simulink model "Simulaciones_Practica2"  (R2021b)
settings: Solver=FixedStepAuto  StartTime=0.0  StopTime=40  FixedStep=0.01  RelTol=1e-3
undefined symbols (not defined in the file or in its folder): b, B, den1, den2, denc, denImp, denR1sim, denR2sim, denR3sim, denR4sim, J, K, k, Kb, Kp, L, m, num1, num2, numc, numImp, numR1sim, numR2sim, numR3sim, numR4sim, R, T, T2
libraries: simulink x9, dspsrcs4 x1
settings Model: Creator=e.delpico.2020  LastModifiedBy=Esther

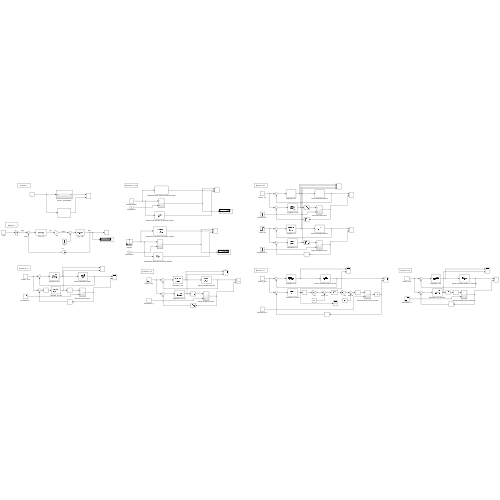
[thumbnail: Simulink's stored preview of the top-level diagram]
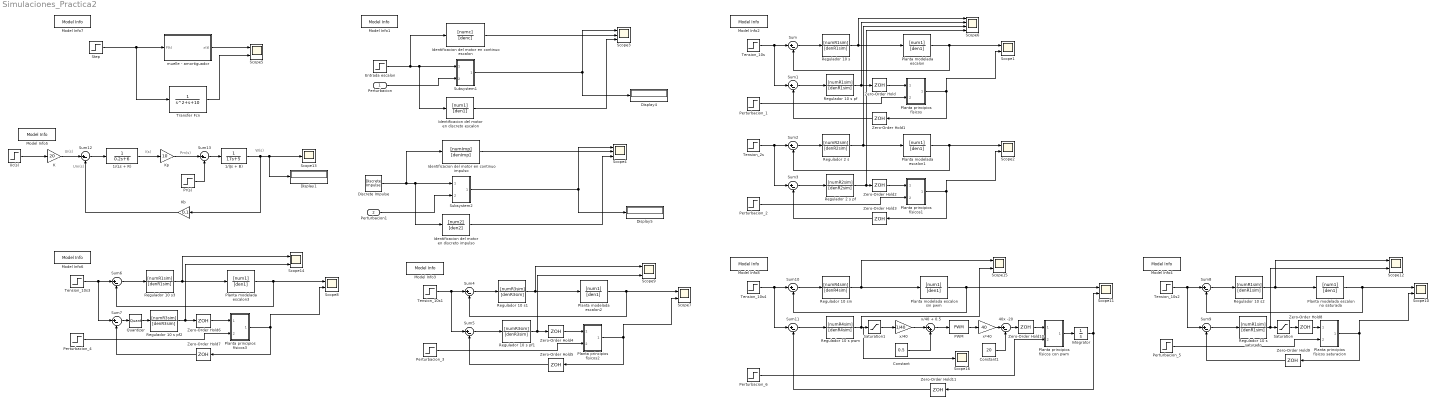
== system Simulaciones_Practica2 ==
  note: Pm(s)
  note: Um(s)
  note: Ui(s)
  note: W(s)
  note: I(s)
  Perturbacion : Inport
  Perturbacion1 : Inport  Port=2
  1/(Js + B) : TransferFcn  Denominator=[17 5]
  1/(Ls + R) : TransferFcn  Denominator=[0.2 6]
  40x -20 : Sum  Inputs=|+-
  Constant : Constant  Value=0.5
  Constant1 : Constant  Value=20
  Discrete Impulse : dspsrcs4/Discrete  Impulse  Delay=0  SampleTime=T  FrameSample=1  OutputFrames=off  dataType=double  isSigned=on  wordLen=16  udDataType=sfix(16)  fracBitsMode=Best precision  numFracBits=15  OutDataTypeStr=double  LastOutDataTypeStr=double
  Display1 : Display
  Display4 : Display
  Display5 : Display
  Entrada escalon : Step  Time=5  SampleTime=0
  Identificacion del motor en continuo escalon : TransferFcn  Numerator=[numc]  Denominator=[denc]
  Identificacion del motor en continuo impulso : TransferFcn  Numerator=[numImp]  Denominator=[denImp]
  Identificacion del motor en discreto escalon : DiscreteTransferFcn  Numerator=[num1]  Denominator=[den1]  SampleTime=T
  Identificacion del motor en discreto impulso : DiscreteTransferFcn  Numerator=[num2]  Denominator=[den2]  SampleTime=T
  Integrator : Integrator
  K : Gain  Gain=20
  Kb : Gain  Gain=0.1
  Kp : Gain  Gain=10
  Model Info1 : simulink/Model-Wide Utilities/Model Info  Frame=on  DisplayStringWithTags=Ejercicio 3.1 a y b  HorizontalTextAlignment=Center  LeftAlignmentValue=0.5
  Model Info2 : simulink/Model-Wide Utilities/Model Info  Frame=on  DisplayStringWithTags=Ejercicio 3.2.3  HorizontalTextAlignment=Center  LeftAlignmentValue=0.5
  Model Info3 : simulink/Model-Wide Utilities/Model Info  Frame=on  DisplayStringWithTags=Ejercicio 4.1.5  HorizontalTextAlignment=Center  LeftAlignmentValue=0.5
  Model Info4 : simulink/Model-Wide Utilities/Model Info  Frame=on  DisplayStringWithTags=Ejercicio 4.1.8  HorizontalTextAlignment=Center  LeftAlignmentValue=0.5
  Model Info5 : simulink/Model-Wide Utilities/Model Info  Frame=on  DisplayStringWithTags=Ejercicio 2  HorizontalTextAlignment=Center  LeftAlignmentValue=0.5
  Model Info6 : simulink/Model-Wide Utilities/Model Info  Frame=on  DisplayStringWithTags=Ejercicio 4.1.4  HorizontalTextAlignment=Center  LeftAlignmentValue=0.5
  Model Info7 : simulink/Model-Wide Utilities/Model Info  Frame=on  DisplayStringWithTags=Ejercicio 1  HorizontalTextAlignment=Center  LeftAlignmentValue=0.5
  Model Info8 : simulink/Model-Wide Utilities/Model Info  Frame=on  DisplayStringWithTags=Ejercicio 4.1.7  HorizontalTextAlignment=Center  LeftAlignmentValue=0.5
  PWM : simulink/Discontinuities/PWM  DisableCoverage=on  Period=1  DisallowZeroDutyCycle=off  RunAtFixedTimeIntervals=on  SampleTime=T
  Perturbacion_{1..4} (4 alike) : Step  Time=15  After=120  SampleTime=0
  Perturbacion_5 : Step  Time=5  After=120  SampleTime=0
  Perturbacion_6 : Step  Time=5  After=120  SampleTime=0
  Planta modelada escalon{,1..3} (4 alike) : DiscreteTransferFcn  Numerator=[num1]  Denominator=[den1]  SampleTime=T
  Planta modelada escalon no saturada : DiscreteTransferFcn  Numerator=[num1]  Denominator=[den1]  SampleTime=T
  Planta modelada escalon sin pwm : DiscreteTransferFcn  Numerator=[num1]  Denominator=[den1]  SampleTime=T
  Planta principios físicos : Subsystem
  Planta principios físicos con pwm : Subsystem
  Planta principios físicos saturacion : Subsystem
  Planta principios físicos1 : Subsystem
  Planta principios físicos2 : Subsystem
  Planta principios físicos3 : Subsystem
  Pr(s) : Step  Time=20  After=120  SampleTime=0
  Quantizer : Quantizer
  Regulador 10 s : DiscreteTransferFcn  Numerator=[numR1sim]  Denominator=[denR1sim]  SampleTime=T
  Regulador 10 s pf : DiscreteTransferFcn  Numerator=[numR1sim]  Denominator=[denR1sim]  SampleTime=T
  Regulador 10 s pf1 : DiscreteTransferFcn  Numerator=[numR3sim]  Denominator=[denR3sim]  SampleTime=T2
  Regulador 10 s pf2 : DiscreteTransferFcn  Numerator=[numR3sim]  Denominator=[denR3sim]  SampleTime=T
  Regulador 10 s pwm : DiscreteTransferFcn  Numerator=[numR4sim]  Denominator=[denR4sim]  SampleTime=T
  Regulador 10 s saturado : DiscreteTransferFcn  Numerator=[numR1sim]  Denominator=[denR1sim]  SampleTime=T
  Regulador 10 s1 : DiscreteTransferFcn  Numerator=[numR3sim]  Denominator=[denR3sim]  SampleTime=T2
  Regulador 10 s2 : DiscreteTransferFcn  Numerator=[numR1sim]  Denominator=[denR1sim]  SampleTime=T
  Regulador 10 s3 : DiscreteTransferFcn  Numerator=[numR1sim]  Denominator=[denR1sim]  SampleTime=T
  Regulador 10 sin : DiscreteTransferFcn  Numerator=[numR4sim]  Denominator=[denR4sim]  SampleTime=T
  Regulador 2 s : DiscreteTransferFcn  Numerator=[numR2sim]  Denominator=[denR2sim]  SampleTime=T
  Regulador 2 s pf : DiscreteTransferFcn  Numerator=[numR2sim]  Denominator=[denR2sim]  SampleTime=T
  Saturation : Saturate  UpperLimit=20  LowerLimit=-20
  Saturation1 : Saturate  UpperLimit=20  LowerLimit=-20  LinearizeAsGain=off
  Scope{1..2,5,7..12,14..15} (11 alike) : Scope  NumInputPorts=2
  Scope13 : Scope
  Scope16 : Scope
  Scope3 : Scope  NumInputPorts=3
  Scope4 : Scope  NumInputPorts=3
  Scope6 : Scope  NumInputPorts=4
  Step : Step  Time=0  SampleTime=0
  Subsystem1 : Subsystem
  Subsystem2 : Subsystem
  Sum{,1..13} (14 alike) : Sum  Inputs=|+-
  Tension_10s{,1,3..4} (4 alike) : Step  Time=5  After=20  SampleTime=0
  Tension_10s2 : Step  Time=5  After=120  SampleTime=0
  Tension_2s : Step  Time=5  After=20  SampleTime=0
  Transfer Fcn : TransferFcn  Denominator=[1 1 10]
  Uc(s) : Step  Time=0  After=20  SampleTime=0
  Zero-Order Hold{,1..3,6..11} (10 alike) : ZeroOrderHold  SampleTime=T
  Zero-Order Hold4 : ZeroOrderHold  SampleTime=T2
  Zero-Order Hold5 : ZeroOrderHold  SampleTime=T2
  muelle - amortiguador : Subsystem
  x*40 : Gain  Gain=40
  x/40 : Gain  Gain=1/40
  x/40 + 0.5 : Sum  Inputs=|++
  wires:
  Subsystem1/1(Out1) -> Scope3/1, Display4/1
  Perturbacion/1 -> Subsystem1/2(In1)
  Entrada escalon/1 -> Identificacion del motor en continuo escalon/1, Identificacion del motor en discreto escalon/1, Subsystem1/1(In2)
  Identificacion del motor en discreto escalon/1 -> Scope3/3
  Identificacion del motor en continuo escalon/1 -> Scope3/2
  Identificacion del motor en continuo impulso/1 -> Scope4/2
  Identificacion del motor en discreto impulso/1 -> Scope4/3
  Subsystem2/1(Out1) -> Scope4/1, Display5/1
  Perturbacion1/1 -> Subsystem2/2(In1)
  Discrete Impulse/1 -> Identificacion del motor en continuo impulso/1, Identificacion del motor en discreto impulso/1, Subsystem2/1(In2)
  Tension_10s/1 -> Sum1/1, Sum/1
  Sum/1 -> Regulador 10 s/1
  Regulador 10 s/1 -> Scope6/1, Planta modelada escalon/1
  Planta modelada escalon/1 -> Scope1/1, Sum/2
  Sum1/1 -> Regulador 10 s pf/1
  Planta principios físicos/1(Out1) -> Scope1/2, Zero-Order Hold1/1
  Regulador 10 s pf/1 -> Scope6/2, Zero-Order Hold/1
  Zero-Order Hold/1 -> Planta principios físicos/1(In2)
  Zero-Order Hold1/1 -> Sum1/2
  Perturbacion_1/1 -> Planta principios físicos/2(In1)
  Perturbacion_2/1 -> Planta principios físicos1/2(In1)
  Planta modelada escalon1/1 -> Sum2/2, Scope2/1
  Regulador 2 s pf/1 -> Scope6/4, Zero-Order Hold2/1
  Sum3/1 -> Regulador 2 s pf/1
  Regulador 2 s/1 -> Planta modelada escalon1/1, Scope6/3
  Zero-Order Hold2/1 -> Planta principios físicos1/1(In2)
  Zero-Order Hold3/1 -> Sum3/2
  Tension_2s/1 -> Sum3/1, Sum2/1
  Sum2/1 -> Regulador 2 s/1
  Planta principios físicos1/1(Out1) -> Scope2/2, Zero-Order Hold3/1
  Step/1 -> Transfer Fcn/1, muelle - amortiguador/1(F(t))
  muelle - amortiguador/1(x(t)) -> Scope5/1
  Transfer Fcn/1 -> Scope5/2
  Planta modelada escalon2/1 -> Scope7/1, Sum4/2
  Planta principios físicos2/1(Out1) -> Scope7/2, Zero-Order Hold5/1
  Sum5/1 -> Regulador 10 s pf1/1
  Regulador 10 s1/1 -> Scope9/1, Planta modelada escalon2/1
  Regulador 10 s pf1/1 -> Scope9/2, Zero-Order Hold4/1
  Zero-Order Hold4/1 -> Planta principios físicos2/1(In2)
  Zero-Order Hold5/1 -> Sum5/2
  Tension_10s1/1 -> Sum5/1, Sum4/1
  Sum4/1 -> Regulador 10 s1/1
  Perturbacion_3/1 -> Planta principios físicos2/2(In1)
  Sum8/1 -> Regulador 10 s2/1
  Perturbacion_5/1 -> Planta principios físicos saturacion/2(In1)
  Tension_10s2/1 -> Sum9/1, Sum8/1
  Zero-Order Hold9/1 -> Sum9/2
  Zero-Order Hold8/1 -> Planta principios físicos saturacion/1(In2)
  Planta principios físicos saturacion/1(Out1) -> Scope10/2, Zero-Order Hold9/1
  Planta modelada escalon no saturada/1 -> Scope10/1, Sum8/2
  Regulador 10 s2/1 -> Scope12/1, Planta modelada escalon no saturada/1
  Sum9/1 -> Regulador 10 s saturado/1
  Regulador 10 s saturado/1 -> Scope12/2, Saturation/1
  Saturation/1 -> Zero-Order Hold8/1
  Kp/1 -> Sum13/1
  K/1 -> Sum12/1
  Uc(s)/1 -> K/1
  Kb/1 -> Sum12/2
  1/(Ls + R)/1 -> Kp/1
  Sum13/1 -> 1/(Js + B)/1
  1/(Js + B)/1 -> Kb/1, Display1/1, Scope13/1
  Sum12/1 -> 1/(Ls + R)/1
  Pr(s)/1 -> Sum13/2
  Sum6/1 -> Regulador 10 s3/1
  Perturbacion_4/1 -> Planta principios físicos3/2(In1)
  Tension_10s3/1 -> Sum7/1, Sum6/1
  Zero-Order Hold7/1 -> Sum7/2
  Zero-Order Hold6/1 -> Planta principios físicos3/1(In2)
  Planta principios físicos3/1(Out1) -> Scope8/2, Zero-Order Hold7/1
  Planta modelada escalon3/1 -> Scope8/1, Sum6/2
  Regulador 10 s3/1 -> Scope14/1, Planta modelada escalon3/1
  Regulador 10 s pf2/1 -> Scope14/2, Zero-Order Hold6/1
  Quantizer/1 -> Regulador 10 s pf2/1
  Sum7/1 -> Quantizer/1
  Sum11/1 -> Regulador 10 s pwm/1
  Regulador 10 sin/1 -> Scope15/1, Planta modelada escalon sin pwm/1
  Planta modelada escalon sin pwm/1 -> Scope11/1, Sum10/2
  Regulador 10 s pwm/1 -> Scope16/1, Scope15/2, Saturation1/1
  Zero-Order Hold11/1 -> Sum11/2
  Perturbacion_6/1 -> Planta principios físicos con pwm/2(In1)
  Zero-Order Hold10/1 -> Planta principios físicos con pwm/1(In2)
  Tension_10s4/1 -> Sum11/1, Sum10/1
  Sum10/1 -> Regulador 10 sin/1
  Saturation1/1 -> x/40/1
  PWM/1 -> x*40/1
  Constant/1 -> x/40 + 0.5/2
  x/40/1 -> x/40 + 0.5/1
  x/40 + 0.5/1 -> PWM/1
  x*40/1 -> 40x -20/1
  40x -20/1 -> Zero-Order Hold10/1
  Constant1/1 -> 40x -20/2
  Planta principios físicos con pwm/1(Out1) -> Integrator/1
  Integrator/1 -> Scope11/2, Zero-Order Hold11/1

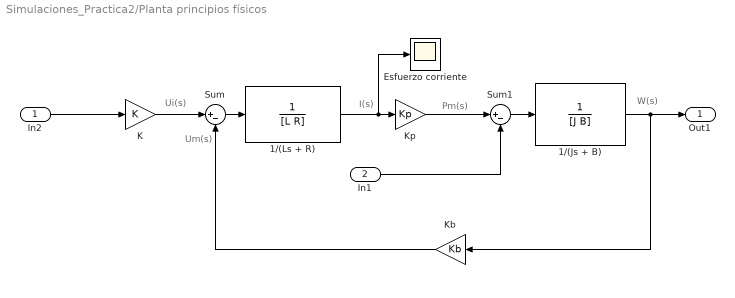
== system Simulaciones_Practica2/Planta principios físicos ==
  note: W(s)
  note: Pm(s)
  note: Um(s)
  note: I(s)
  note: Ui(s)
  In2 : Inport
  In1 : Inport  Port=2
  1/(Js + B) : TransferFcn  Denominator=[J B]
  1/(Ls + R) : TransferFcn  Denominator=[L R]
  Esfuerzo corriente : Scope
  K : Gain  Gain=K
  Kb : Gain  Gain=Kb
  Kp : Gain  Gain=Kp
  Sum : Sum  Inputs=|+-
  Sum1 : Sum  Inputs=|+-
  Out1 : Outport
  wires:
  1/(Js + B)/1 -> Out1/1, Kb/1
  Kb/1 -> Sum/2
  Sum/1 -> 1/(Ls + R)/1
  K/1 -> Sum/1
  Sum1/1 -> 1/(Js + B)/1
  1/(Ls + R)/1 -> Esfuerzo corriente/1, Kp/1
  Kp/1 -> Sum1/1
  In2/1 -> K/1
  In1/1 -> Sum1/2

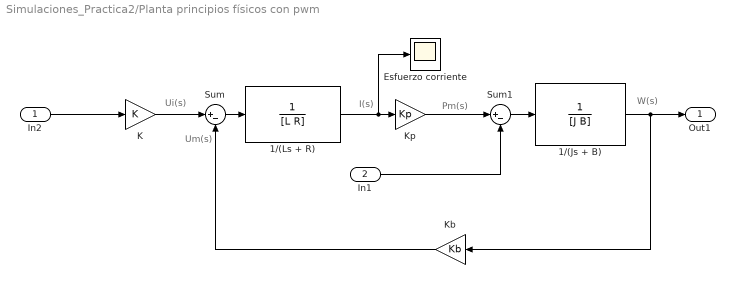
== system Simulaciones_Practica2/Planta principios físicos con pwm ==
  note: W(s)
  note: Pm(s)
  note: Um(s)
  note: I(s)
  note: Ui(s)
  In2 : Inport
  In1 : Inport  Port=2
  1/(Js + B) : TransferFcn  Denominator=[J B]
  1/(Ls + R) : TransferFcn  Denominator=[L R]
  Esfuerzo corriente : Scope
  K : Gain  Gain=K
  Kb : Gain  Gain=Kb
  Kp : Gain  Gain=Kp
  Sum : Sum  Inputs=|+-
  Sum1 : Sum  Inputs=|+-
  Out1 : Outport
  wires:
  1/(Js + B)/1 -> Out1/1, Kb/1
  Kb/1 -> Sum/2
  Sum/1 -> 1/(Ls + R)/1
  K/1 -> Sum/1
  Sum1/1 -> 1/(Js + B)/1
  1/(Ls + R)/1 -> Esfuerzo corriente/1, Kp/1
  Kp/1 -> Sum1/1
  In2/1 -> K/1
  In1/1 -> Sum1/2

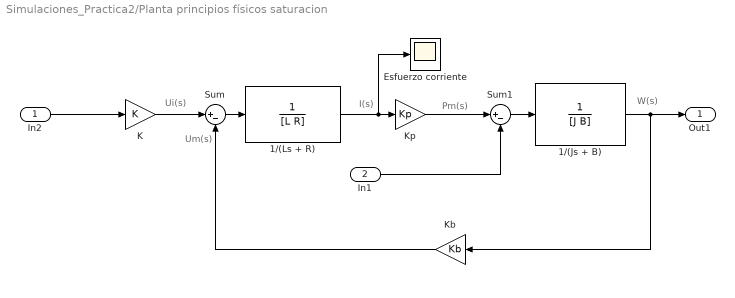
== system Simulaciones_Practica2/Planta principios físicos saturacion ==
  note: W(s)
  note: Pm(s)
  note: Um(s)
  note: I(s)
  note: Ui(s)
  In2 : Inport
  In1 : Inport  Port=2
  1/(Js + B) : TransferFcn  Denominator=[J B]
  1/(Ls + R) : TransferFcn  Denominator=[L R]
  Esfuerzo corriente : Scope
  K : Gain  Gain=K
  Kb : Gain  Gain=Kb
  Kp : Gain  Gain=Kp
  Sum : Sum  Inputs=|+-
  Sum1 : Sum  Inputs=|+-
  Out1 : Outport
  wires:
  1/(Js + B)/1 -> Out1/1, Kb/1
  Kb/1 -> Sum/2
  Sum/1 -> 1/(Ls + R)/1
  K/1 -> Sum/1
  Sum1/1 -> 1/(Js + B)/1
  1/(Ls + R)/1 -> Esfuerzo corriente/1, Kp/1
  Kp/1 -> Sum1/1
  In2/1 -> K/1
  In1/1 -> Sum1/2

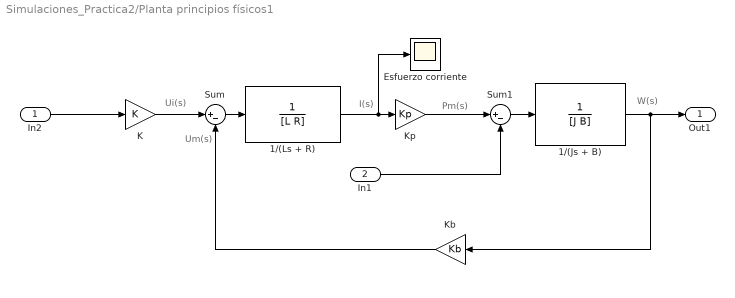
== system Simulaciones_Practica2/Planta principios físicos1 ==
  note: W(s)
  note: Pm(s)
  note: Um(s)
  note: I(s)
  note: Ui(s)
  In2 : Inport
  In1 : Inport  Port=2
  1/(Js + B) : TransferFcn  Denominator=[J B]
  1/(Ls + R) : TransferFcn  Denominator=[L R]
  Esfuerzo corriente : Scope
  K : Gain  Gain=K
  Kb : Gain  Gain=Kb
  Kp : Gain  Gain=Kp
  Sum : Sum  Inputs=|+-
  Sum1 : Sum  Inputs=|+-
  Out1 : Outport
  wires:
  1/(Js + B)/1 -> Out1/1, Kb/1
  Kb/1 -> Sum/2
  Sum/1 -> 1/(Ls + R)/1
  K/1 -> Sum/1
  Sum1/1 -> 1/(Js + B)/1
  1/(Ls + R)/1 -> Esfuerzo corriente/1, Kp/1
  Kp/1 -> Sum1/1
  In2/1 -> K/1
  In1/1 -> Sum1/2

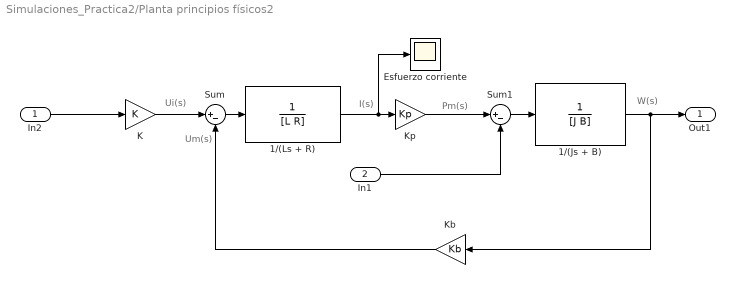
== system Simulaciones_Practica2/Planta principios físicos2 ==
  note: W(s)
  note: Pm(s)
  note: Um(s)
  note: I(s)
  note: Ui(s)
  In2 : Inport
  In1 : Inport  Port=2
  1/(Js + B) : TransferFcn  Denominator=[J B]
  1/(Ls + R) : TransferFcn  Denominator=[L R]
  Esfuerzo corriente : Scope
  K : Gain  Gain=K
  Kb : Gain  Gain=Kb
  Kp : Gain  Gain=Kp
  Sum : Sum  Inputs=|+-
  Sum1 : Sum  Inputs=|+-
  Out1 : Outport
  wires:
  1/(Js + B)/1 -> Out1/1, Kb/1
  Kb/1 -> Sum/2
  Sum/1 -> 1/(Ls + R)/1
  K/1 -> Sum/1
  Sum1/1 -> 1/(Js + B)/1
  1/(Ls + R)/1 -> Esfuerzo corriente/1, Kp/1
  Kp/1 -> Sum1/1
  In2/1 -> K/1
  In1/1 -> Sum1/2

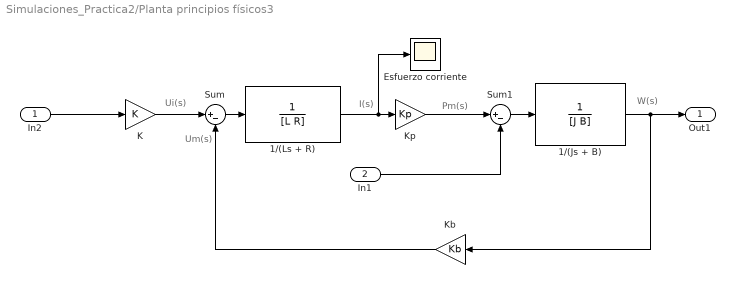
== system Simulaciones_Practica2/Planta principios físicos3 ==
  note: W(s)
  note: Pm(s)
  note: Um(s)
  note: I(s)
  note: Ui(s)
  In2 : Inport
  In1 : Inport  Port=2
  1/(Js + B) : TransferFcn  Denominator=[J B]
  1/(Ls + R) : TransferFcn  Denominator=[L R]
  Esfuerzo corriente : Scope
  K : Gain  Gain=K
  Kb : Gain  Gain=Kb
  Kp : Gain  Gain=Kp
  Sum : Sum  Inputs=|+-
  Sum1 : Sum  Inputs=|+-
  Out1 : Outport
  wires:
  1/(Js + B)/1 -> Out1/1, Kb/1
  Kb/1 -> Sum/2
  Sum/1 -> 1/(Ls + R)/1
  K/1 -> Sum/1
  Sum1/1 -> 1/(Js + B)/1
  1/(Ls + R)/1 -> Esfuerzo corriente/1, Kp/1
  Kp/1 -> Sum1/1
  In2/1 -> K/1
  In1/1 -> Sum1/2

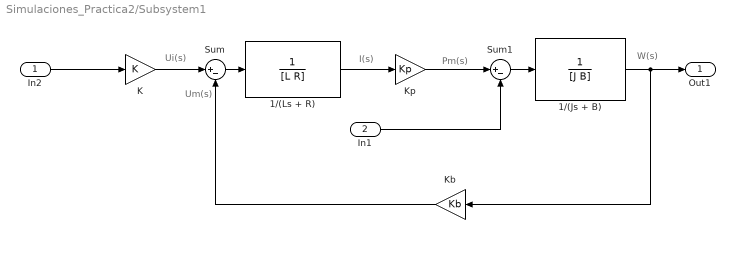
== system Simulaciones_Practica2/Subsystem1 ==
  note: W(s)
  note: Pm(s)
  note: Um(s)
  note: I(s)
  note: Ui(s)
  In2 : Inport
  In1 : Inport  Port=2
  1/(Js + B) : TransferFcn  Denominator=[J B]
  1/(Ls + R) : TransferFcn  Denominator=[L R]
  K : Gain  Gain=K
  Kb : Gain  Gain=Kb
  Kp : Gain  Gain=Kp
  Sum : Sum  Inputs=|+-
  Sum1 : Sum  Inputs=|+-
  Out1 : Outport
  wires:
  1/(Js + B)/1 -> Out1/1, Kb/1
  Kb/1 -> Sum/2
  Sum/1 -> 1/(Ls + R)/1
  K/1 -> Sum/1
  Sum1/1 -> 1/(Js + B)/1
  1/(Ls + R)/1 -> Kp/1
  Kp/1 -> Sum1/1
  In2/1 -> K/1
  In1/1 -> Sum1/2

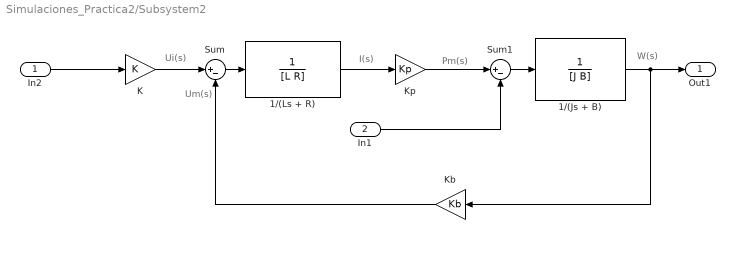
== system Simulaciones_Practica2/Subsystem2 ==
  note: W(s)
  note: Pm(s)
  note: Um(s)
  note: I(s)
  note: Ui(s)
  In2 : Inport
  In1 : Inport  Port=2
  1/(Js + B) : TransferFcn  Denominator=[J B]
  1/(Ls + R) : TransferFcn  Denominator=[L R]
  K : Gain  Gain=K
  Kb : Gain  Gain=Kb
  Kp : Gain  Gain=Kp
  Sum : Sum  Inputs=|+-
  Sum1 : Sum  Inputs=|+-
  Out1 : Outport
  wires:
  1/(Js + B)/1 -> Out1/1, Kb/1
  Kb/1 -> Sum/2
  Sum/1 -> 1/(Ls + R)/1
  K/1 -> Sum/1
  Sum1/1 -> 1/(Js + B)/1
  1/(Ls + R)/1 -> Kp/1
  Kp/1 -> Sum1/1
  In2/1 -> K/1
  In1/1 -> Sum1/2

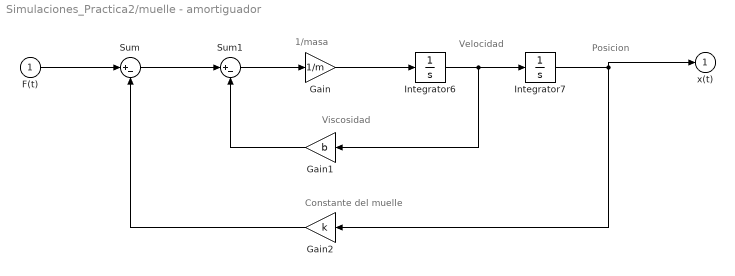
== system Simulaciones_Practica2/muelle - amortiguador ==
  note: 1/masa
  note: Velocidad
  note: Posicion
  note: Viscosidad
  note: Constante del muelle
  F(t) : Inport
  Gain : Gain  Gain=1/m
  Gain1 : Gain  Gain=b
  Gain2 : Gain  Gain=k
  Integrator6 : Integrator
  Integrator7 : Integrator
  Sum : Sum  Inputs=|+-
  Sum1 : Sum  Inputs=|+-
  x(t) : Outport
  wires:
  Gain1/1 -> Sum1/2
  Sum/1 -> Sum1/1
  Integrator7/1 -> x(t)/1, Gain2/1
  Gain/1 -> Integrator6/1
  Integrator6/1 -> Gain1/1, Integrator7/1
  F(t)/1 -> Sum/1
  Sum1/1 -> Gain/1
  Gain2/1 -> Sum/2
